simulink model "monitor"  (R2024a)
settings: Solver=VariableStepAuto  StartTime=0.0  StopTime=inf  RelTol=1e-3
libraries: instrumentseriallib x2
settings Model: Creator=alexivanov  LastModifiedBy=alexivanov

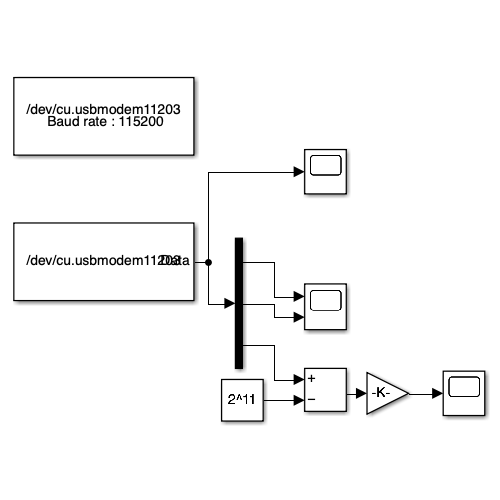
[thumbnail: Simulink's stored preview of the top-level diagram]
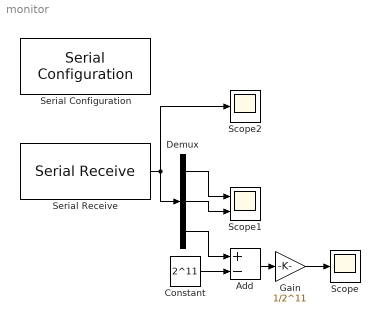
== system monitor ==
  Add : Sum  Inputs=+-
  Constant : Constant  Value=2^11
  Demux : Demux  Outputs=3
  Gain : Gain  Gain=1/2^11
  Scope : Scope
  Scope1 : Scope  NumInputPorts=2
  Scope2 : Scope
  Serial Configuration : instrumentseriallib/Serial Configuration  Priority=-200000  PortSel=/dev/cu.usbmodem11203  Port=/dev/cu.usbmodem11203  ComPort=/dev/cu.usbmodem11203  BaudRate=115200  DataBits=8  Parity=none  StopBits=1  ByteOrder=little-endian  FlowControl=none  Timeout=10  SimulateUsing=Interpreted execution  BlockInModel=on  aMode=1
  Serial Receive : instrumentseriallib/Serial Receive  Priority=1  PortSel=/dev/cu.usbmodem11203  Port=/dev/cu.usbmodem11203  ComPort=/dev/cu.usbmodem11203  DataType=uint16  SaveDataType=uint8  ToggleHeader=on  Header=[205 171]  ToggleDataSize=on  DataSize=[3 1]  ToggleTerminator=on  Terminator=Custom terminator  CustomTerminator=[218 190]  InputFormat=Column major  EnableBlockingMode=on  ActionDataUnavailable=Output last received value  ActionWhenDataUnavailable=Output last received value  CustomValue=0  SampleTime=0.001  SimulateUsing=Interpreted execution  BlockInModel=on  aMode=1
  wires:
  Serial Receive/1 -> Scope2/1, Demux/1
  Demux/2 -> Scope1/2
  Demux/3 -> Add/1
  Constant/1 -> Add/2
  Add/1 -> Gain/1
  Gain/1 -> Scope/1
  Demux/1 -> Scope1/1
